simulink model "NFBLB_HYP_NON_LIN"  (R2022b)
settings: Solver=VariableStepAuto  StartTime=0.0  StopTime=90  RelTol=1e-3
model workspace (MATLAB code in the model file):
  | Kab=12;
  | Kca=16;
  | Fb=2;
  | Kbc=8;
  | Kcb=10;
  | Kia=8;
  | Fa=6;
  | x_star=[0.4;0.64;0.5];
settings Model: Creator=priya  LastModifiedBy=pxb271
settings SolverCC: AlgebraicLoopSolver=TrustRegion
settings DebuggingCC: UnconnectedInputMsg=warning  UnconnectedOutputMsg=warning  UnconnectedLineMsg=warning  SFMachineParentedDataDiag=warning
settings ModelReferenceCC: EnableRefExpFcnMdlSchedulingChecks=on
settings RTWCC: DLArmComputeVersion=19.05

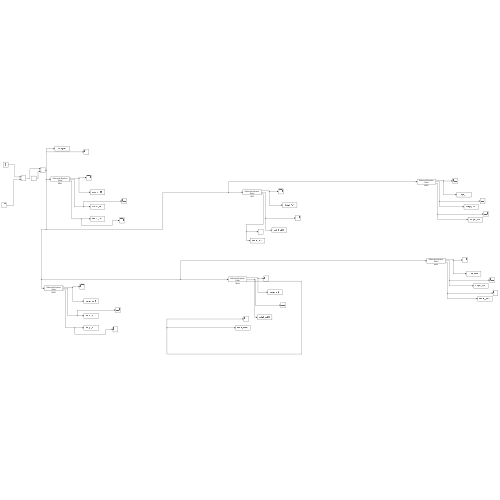
[thumbnail: Simulink's stored preview of the top-level diagram]
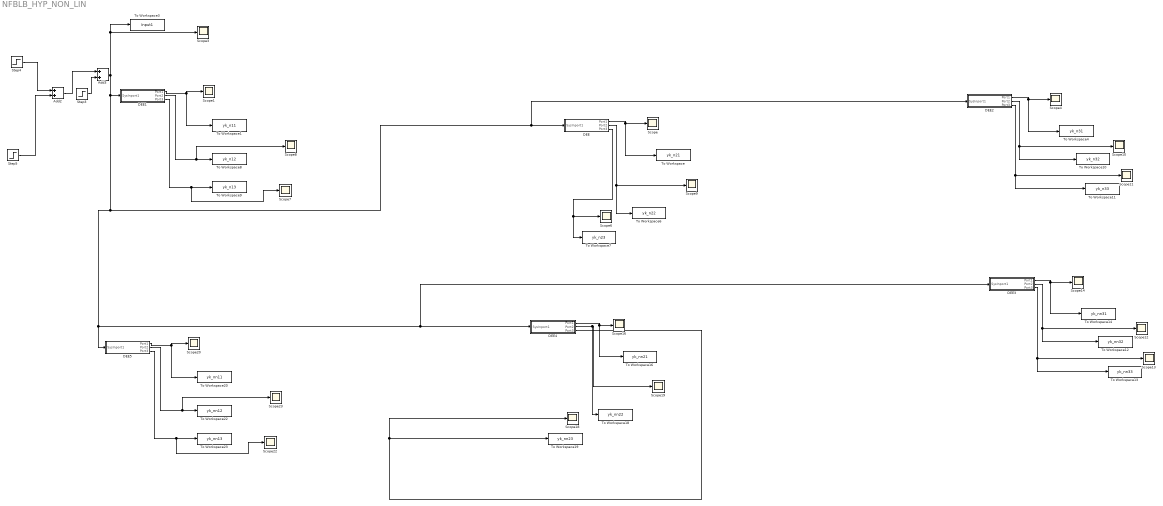
== system NFBLB_HYP_NON_LIN ==
  Add2 : Sum
  Add3 : Sum
  DEE : Subsystem  mask(Differential Equation Editor (DEE)){}
      settings: OpenFcn=diffeqed
      mask Display: disp('Differential Equation\n Editor')
  DEE1 : Subsystem  mask(Differential Equation Editor (DEE)){}
      settings: OpenFcn=diffeqed
      mask Display: disp('Differential Equation\n Editor')
  DEE2 : Subsystem  mask(Differential Equation Editor (DEE)){}
      settings: OpenFcn=diffeqed
      mask Display: disp('Differential Equation\n Editor')
  DEE3 : Subsystem  mask(Differential Equation Editor (DEE)){}
      settings: OpenFcn=diffeqed
      mask Display: disp('Differential Equation\n Editor')
  DEE4 : Subsystem  mask(Differential Equation Editor (DEE)){}
      settings: OpenFcn=diffeqed
      mask Display: disp('Differential Equation\n Editor')
  DEE5 : Subsystem  mask(Differential Equation Editor (DEE)){}
      settings: OpenFcn=diffeqed
      mask Display: disp('Differential Equation\n Editor')
  Scope{,1,3..4,6..14,16,18..20,22..23} (19 alike) : Scope
  Step3 : Step  Time=50  After=0.15  SampleTime=0
  Step4 : Step  Time=5  After=0.5  SampleTime=0
  Step5 : Step  Time=25  After=0.2  SampleTime=0
  To Workspace : ToWorkspace  VariableName=yk_n21  SampleTime=-1
  To Workspace1 : ToWorkspace  VariableName=yk_n11  SampleTime=-1
  To Workspace10 : ToWorkspace  VariableName=yk_n32  SampleTime=-1
  To Workspace11 : ToWorkspace  VariableName=yk_n33  SampleTime=-1
  To Workspace12 : ToWorkspace  VariableName=yk_nn32  SampleTime=-1
  To Workspace13 : ToWorkspace  VariableName=yk_nn33  SampleTime=-1
  To Workspace14 : ToWorkspace  VariableName=yk_nn31  SampleTime=-1
  To Workspace16 : ToWorkspace  VariableName=yk_nn21  SampleTime=-1
  To Workspace18 : ToWorkspace  VariableName=yk_nn22  SampleTime=-1
  To Workspace19 : ToWorkspace  VariableName=yk_nn23  SampleTime=-1
  To Workspace20 : ToWorkspace  VariableName=yk_nn11  SampleTime=-1
  To Workspace22 : ToWorkspace  VariableName=yk_nn12  SampleTime=-1
  To Workspace23 : ToWorkspace  VariableName=yk_nn13  SampleTime=-1
  To Workspace3 : ToWorkspace  VariableName=Input1  SampleTime=-1
  To Workspace4 : ToWorkspace  VariableName=yk_n31  SampleTime=-1
  To Workspace6 : ToWorkspace  VariableName=yk_n22  SampleTime=-1
  To Workspace7 : ToWorkspace  VariableName=yk_n23  SampleTime=-1
  To Workspace8 : ToWorkspace  VariableName=yk_n12  SampleTime=-1
  To Workspace9 : ToWorkspace  VariableName=yk_n13  SampleTime=-1
  wires:
  DEE2/1(Port1) -> To Workspace4/1, Scope4/1
  Step5/1 -> Add2/2
  DEE1/1(Port1) -> To Workspace1/1, Scope1/1
  Add3/1 -> Scope3/1, To Workspace3/1, DEE3/1(SysInport1), DEE4/1(SysInport1), DEE5/1(SysInport1), DEE2/1(SysInport1), DEE/1(SysInport1), DEE1/1(SysInport1)
  Step3/1 -> Add3/2
  Step4/1 -> Add2/1
  DEE/3(Port3) -> Scope6/1, To Workspace7/1
  DEE1/3(Port3) -> Scope7/1, To Workspace9/1
  DEE/1(Port1) -> To Workspace/1, Scope/1
  DEE1/2(Port2) -> Scope8/1, To Workspace8/1
  DEE/2(Port2) -> To Workspace6/1, Scope9/1
  Add2/1 -> Add3/1
  DEE2/2(Port2) -> To Workspace10/1, Scope10/1
  DEE2/3(Port3) -> To Workspace11/1, Scope11/1
  DEE3/1(Port1) -> To Workspace14/1, Scope14/1
  DEE3/3(Port3) -> To Workspace13/1, Scope13/1
  DEE3/2(Port2) -> To Workspace12/1, Scope12/1
  DEE4/1(Port1) -> To Workspace16/1, Scope16/1
  DEE4/2(Port2) -> To Workspace18/1, Scope19/1
  DEE4/3(Port3) -> Scope18/1, To Workspace19/1
  DEE5/2(Port2) -> Scope23/1, To Workspace22/1
  DEE5/1(Port1) -> To Workspace20/1, Scope20/1
  DEE5/3(Port3) -> Scope22/1, To Workspace23/1

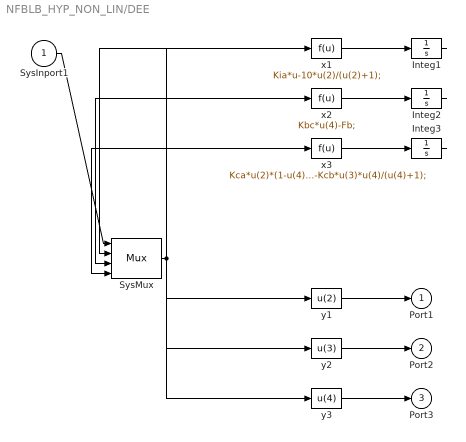
== system NFBLB_HYP_NON_LIN/DEE ==
  SysInport1 : Inport
  Integ1 : Integrator  InitialCondition=x_star(1)
  Integ2 : Integrator  InitialCondition=x_star(2)
  Integ3 : Integrator  InitialCondition=x_star(3)
  SysMux : Mux
  x1 : Fcn  Expr=Kia*u-10*u(2)/(u(2)+1);
  x2 : Fcn  Expr=Kbc*u(4)-Fb;
  x3 : Fcn  Expr=Kca*u(2)*(1-u(4))/(2-u(4))-Kcb*u(3)*u(4)/(u(4)+1);
  y1 : Fcn  Expr=u(2)
  y2 : Fcn  Expr=u(3)
  y3 : Fcn  Expr=u(4)
  Port1 : Outport
  Port2 : Outport  Port=2
  Port3 : Outport  Port=3
  wires:
  SysInport1/1 -> SysMux/1
  SysMux/1 -> x1/1, x2/1, x3/1, y1/1, y2/1, y3/1
  x1/1 -> Integ1/1
  Integ1/1 -> SysMux/2
  x2/1 -> Integ2/1
  Integ2/1 -> SysMux/3
  x3/1 -> Integ3/1
  Integ3/1 -> SysMux/4
  y1/1 -> Port1/1
  y2/1 -> Port2/1
  y3/1 -> Port3/1

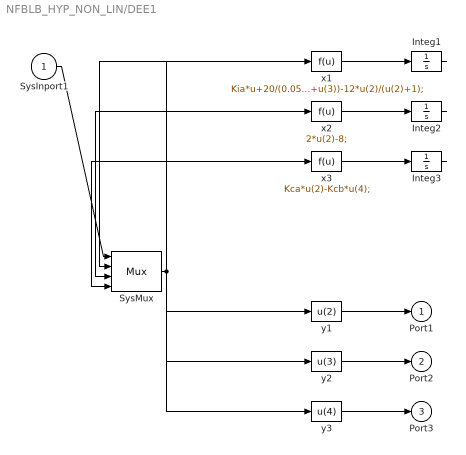
== system NFBLB_HYP_NON_LIN/DEE1 ==
  SysInport1 : Inport
  Integ1 : Integrator
  Integ2 : Integrator
  Integ3 : Integrator
  SysMux : Mux
  x1 : Fcn  Expr=Kia*u+20/(0.05+u(3))-12*u(2)/(u(2)+1);
  x2 : Fcn  Expr=2*u(2)-8;
  x3 : Fcn  Expr=Kca*u(2)-Kcb*u(4);
  y1 : Fcn  Expr=u(2)
  y2 : Fcn  Expr=u(3)
  y3 : Fcn  Expr=u(4)
  Port1 : Outport
  Port2 : Outport  Port=2
  Port3 : Outport  Port=3
  wires:
  SysInport1/1 -> SysMux/1
  SysMux/1 -> x1/1, x2/1, x3/1, y1/1, y2/1, y3/1
  x1/1 -> Integ1/1
  Integ1/1 -> SysMux/2
  x2/1 -> Integ2/1
  Integ2/1 -> SysMux/3
  x3/1 -> Integ3/1
  Integ3/1 -> SysMux/4
  y1/1 -> Port1/1
  y2/1 -> Port2/1
  y3/1 -> Port3/1

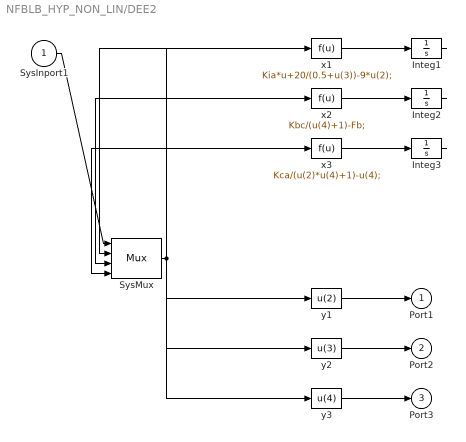
== system NFBLB_HYP_NON_LIN/DEE2 ==
  SysInport1 : Inport
  Integ1 : Integrator  InitialCondition=0.6
  Integ2 : Integrator  InitialCondition=0.5
  Integ3 : Integrator  InitialCondition=3
  SysMux : Mux
  x1 : Fcn  Expr=Kia*u+20/(0.5+u(3))-9*u(2);
  x2 : Fcn  Expr=Kbc/(u(4)+1)-Fb;
  x3 : Fcn  Expr=Kca/(u(2)*u(4)+1)-u(4);
  y1 : Fcn  Expr=u(2)
  y2 : Fcn  Expr=u(3)
  y3 : Fcn  Expr=u(4)
  Port1 : Outport
  Port2 : Outport  Port=2
  Port3 : Outport  Port=3
  wires:
  SysInport1/1 -> SysMux/1
  SysMux/1 -> x1/1, x2/1, x3/1, y1/1, y2/1, y3/1
  x1/1 -> Integ1/1
  Integ1/1 -> SysMux/2
  x2/1 -> Integ2/1
  Integ2/1 -> SysMux/3
  x3/1 -> Integ3/1
  Integ3/1 -> SysMux/4
  y1/1 -> Port1/1
  y2/1 -> Port2/1
  y3/1 -> Port3/1

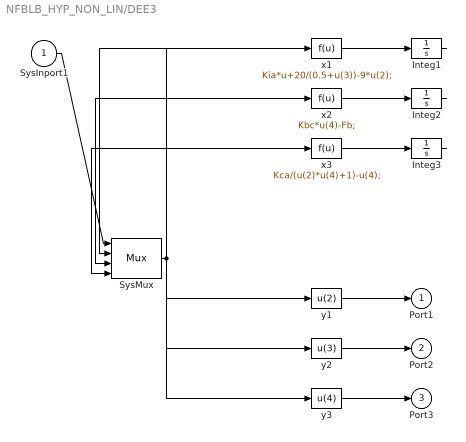
== system NFBLB_HYP_NON_LIN/DEE3 ==
  SysInport1 : Inport
  Integ1 : Integrator  InitialCondition=0.6
  Integ2 : Integrator  InitialCondition=0.5
  Integ3 : Integrator  InitialCondition=3
  SysMux : Mux
  x1 : Fcn  Expr=Kia*u+20/(0.5+u(3))-9*u(2);
  x2 : Fcn  Expr=Kbc*u(4)-Fb;
  x3 : Fcn  Expr=Kca/(u(2)*u(4)+1)-u(4);
  y1 : Fcn  Expr=u(2)
  y2 : Fcn  Expr=u(3)
  y3 : Fcn  Expr=u(4)
  Port1 : Outport
  Port2 : Outport  Port=2
  Port3 : Outport  Port=3
  wires:
  SysInport1/1 -> SysMux/1
  SysMux/1 -> x1/1, x2/1, x3/1, y1/1, y2/1, y3/1
  x1/1 -> Integ1/1
  Integ1/1 -> SysMux/2
  x2/1 -> Integ2/1
  Integ2/1 -> SysMux/3
  x3/1 -> Integ3/1
  Integ3/1 -> SysMux/4
  y1/1 -> Port1/1
  y2/1 -> Port2/1
  y3/1 -> Port3/1

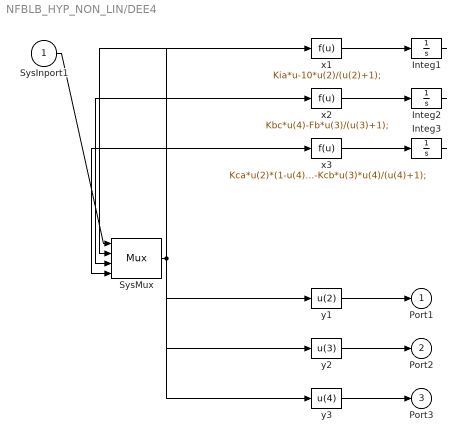
== system NFBLB_HYP_NON_LIN/DEE4 ==
  SysInport1 : Inport
  Integ1 : Integrator  InitialCondition=x_star(1)
  Integ2 : Integrator  InitialCondition=x_star(2)
  Integ3 : Integrator
  SysMux : Mux
  x1 : Fcn  Expr=Kia*u-10*u(2)/(u(2)+1);
  x2 : Fcn  Expr=Kbc*u(4)-Fb*u(3)/(u(3)+1);
  x3 : Fcn  Expr=Kca*u(2)*(1-u(4))/(2-u(4))-Kcb*u(3)*u(4)/(u(4)+1);
  y1 : Fcn  Expr=u(2)
  y2 : Fcn  Expr=u(3)
  y3 : Fcn  Expr=u(4)
  Port1 : Outport
  Port2 : Outport  Port=2
  Port3 : Outport  Port=3
  wires:
  SysInport1/1 -> SysMux/1
  SysMux/1 -> x1/1, x2/1, x3/1, y1/1, y2/1, y3/1
  x1/1 -> Integ1/1
  Integ1/1 -> SysMux/2
  x2/1 -> Integ2/1
  Integ2/1 -> SysMux/3
  x3/1 -> Integ3/1
  Integ3/1 -> SysMux/4
  y1/1 -> Port1/1
  y2/1 -> Port2/1
  y3/1 -> Port3/1

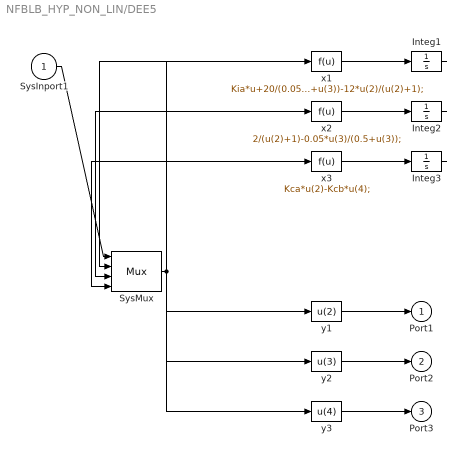
== system NFBLB_HYP_NON_LIN/DEE5 ==
  SysInport1 : Inport
  Integ1 : Integrator
  Integ2 : Integrator
  Integ3 : Integrator
  SysMux : Mux
  x1 : Fcn  Expr=Kia*u+20/(0.05+u(3))-12*u(2)/(u(2)+1);
  x2 : Fcn  Expr=2/(u(2)+1)-0.05*u(3)/(0.5+u(3));
  x3 : Fcn  Expr=Kca*u(2)-Kcb*u(4);
  y1 : Fcn  Expr=u(2)
  y2 : Fcn  Expr=u(3)
  y3 : Fcn  Expr=u(4)
  Port1 : Outport
  Port2 : Outport  Port=2
  Port3 : Outport  Port=3
  wires:
  SysInport1/1 -> SysMux/1
  SysMux/1 -> x1/1, x2/1, x3/1, y1/1, y2/1, y3/1
  x1/1 -> Integ1/1
  Integ1/1 -> SysMux/2
  x2/1 -> Integ2/1
  Integ2/1 -> SysMux/3
  x3/1 -> Integ3/1
  Integ3/1 -> SysMux/4
  y1/1 -> Port1/1
  y2/1 -> Port2/1
  y3/1 -> Port3/1
